simulink model "a2at"  (R2018a)
settings: Solver=ode3  StartTime=0  StopTime=50  FixedStep=Ts  RelTol=1e-3  EnableMultiTasking=on
undefined symbols (not defined in the file): d2r, Earth, ft, initPosLLA, m, mass, s, sigbuilder_block, Ts, Vehicle, WGS84
libraries: simulink x8, aerolibconvert2 x4, aerolibanimutils x2, aerolibfltsims x2, aerolibutil x2, shared6dof x1, aerolibtransform2 x1, vrlib x1, dspswit3 x1
(part 2 of 2)

== matlab function a2at/controll/Subsystem1/MATLAB Function ==
  data: u input; y output
function y = Torque2surface(u)
A=0.349;
u_1=u(1);
u_2=u(2);
u_3=u(3);
yaw_allowance=[0;0;0];
d=[0;0];
yaw_allowance(1)=A-abs(u_1);
yaw_allowance(2)=A-abs(u_2);
yaw_allowance(3)=2*(yaw_allowance(1)+yaw_allowance(2));    
yaw_sign=sign(u_3);
if  yaw_allowance(1)<yaw_allowance(2)   
    if abs(u_3)<2*yaw_allowance(1)   
        d(1)=0.5*u_3;
        d(2)=0.5*u_3;   
    elseif abs(u_3)>yaw_allowance(3)  
        d(1)=yaw_sign*yaw_allowance(1);
        d(2)=yaw_sign*yaw_allowance(2);   
    else  
        d(1)=yaw_sign*yaw_allowance(1);
        d(2)=yaw_sign*(abs(u_3)-yaw_allowance(1));
    end
else
    if abs(u_3)<2*yaw_allowance(2)   
        d(1)=0.5*u_3;
        d(2)=0.5*u_3; 
    elseif abs(u_3)>yaw_allowance(3)
        d(1)=yaw_sign*yaw_allowance(1);
        d(2)=yaw_sign*yaw_allowance(2);  
    else
        d(1)=yaw_sign*(abs(u_3)-yaw_allowance(2));
        d(2)=yaw_sign*yaw_allowance(2);
    end
end
c1=-u_1+d(1);
c2=-u_2+d(2);
c3= u_1+d(1);
c4= u_2+d(2);
y = [c1;c2;c3;c4];

== matlab function a2at/controll/MATLAB Function2 ==
  data: at input; speed output
function speed = at2speed(at)
g=9.788;
HOVER_SPEED = 1225;
K=HOVER_SPEED^2/g;
speed=sqrt((-at)*K);

== matlab function a2at/controll/MATLAB Function3 ==
  data: roll input; pitch input; a input; at output
function at = a2at(roll,pitch,a)
g=9.788;
a_t=a-g;
cosr=cos(roll)*cos(pitch);
cosr=Constrain(cosr,0,pi);
at = a_t/cosr;
